simulink model "laplace_transform"  (R2020a)
settings: Solver=VariableStepAuto  StartTime=0.0  StopTime=10.0  RelTol=1e-3
values from neighbouring files (symbols this model uses):
  Kt = 3.575e-5    (= 3.575e-05)    [main.m]
  M = 1    [main.m]
  omega_0 = sqrt(G*M/Kt)    [main.m]
  u_0 = omega_0    [main.m]
  Z0 = 2    [main.m]
undefined symbols (not defined in the file or in its folder): i
settings Model: Creator=josem  LastModifiedBy=josem

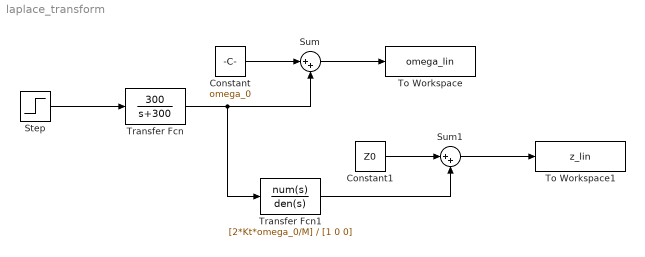
== system laplace_transform ==
  Constant : Constant  Value=omega_0
  Constant1 : Constant  Value=Z0
  Step : Step  After=u(i)-u_0  SampleTime=0
  Sum : Sum  Inputs=|++
  Sum1 : Sum  Inputs=|++
  To Workspace : ToWorkspace  VariableName=omega_lin  SaveFormat=Structure With Time  SampleTime=-1
  To Workspace1 : ToWorkspace  VariableName=z_lin  SaveFormat=Structure With Time  SampleTime=-1
  Transfer Fcn : TransferFcn  Numerator=[300]  Denominator=[1 300]
  Transfer Fcn1 : TransferFcn  Numerator=[2*Kt*omega_0/M]  Denominator=[1 0 0]
  wires:
  Step/1 -> Transfer Fcn/1
  Transfer Fcn/1 -> Sum/2, Transfer Fcn1/1
  Sum/1 -> To Workspace/1
  Constant/1 -> Sum/1
  Constant1/1 -> Sum1/1
  Transfer Fcn1/1 -> Sum1/2
  Sum1/1 -> To Workspace1/1
